simulink model "serialtest"  (Simulink 7.1)
settings: Solver=FixedStepDiscrete  StartTime=0.0  StopTime=10.0  RelTol=1e-3
values from neighbouring files (symbols this model uses):
  count = count+1    (= 2)    [findVI.m]
libraries: xpclib x4, simulink x1
settings Model: Creator=Administrator  LastModifiedBy=jporter  BufferReuse=off
settings DataIOCC: LimitDataPoints=off  SaveTime=off
settings OptimizationCC: BlockReduction=off  OptimizeBlockIOStorage=off  BufferReuse=off  ExpressionFolding=off  LocalBlockOutputs=off
settings HardwareCC: ProdIntDivRoundTo=Zero  ProdEndianess=LittleEndian  ProdHWDeviceType=Generic->32-bit x86 compatible
settings RTWCC: SystemTargetFile=xpctarget.tlc  TemplateMakefile=xpc_default_tmf  Description=xPC Target  ProcessScript=xpctarget_make_rtw_hook
settings xpcTargetCC: TargetFcnLib=ansi_tfl_table_tmw.mat  TargetFunctionLibrary=ANSI_C  CompOptLevelCompliant=off  PortableWordSizes=off  xPCisDownloadable=off

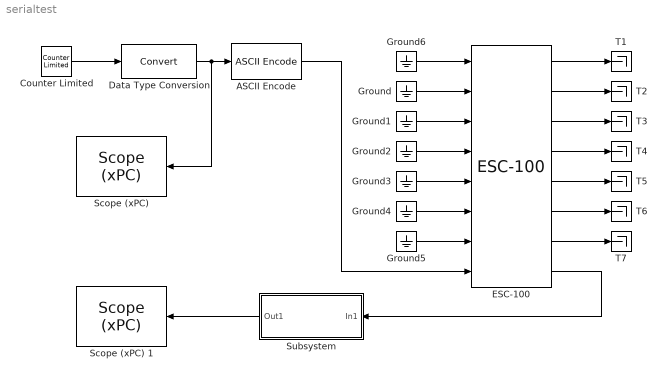
== system serialtest ==
  "ASCII Encode " : xpclib/RS232/ASCII Encode   format=%e\r  nvars=1  maxlength=128  vartypes={'double'}
  Counter Limited : simulink/Sources/Counter Limited  SystemSampleTime=-1  uplimit=99  tsamp=1
  Data Type Conversion : DataTypeConversion  OutDataType=sfix(16)  OutScaling=2^0
  ESC-100 : xpclib/RS232/Quatech/ESC-100/ESC-100  SystemSampleTime=-1  group=Basic Setup  port=8  irqnum=10  slot=[3,6]  baud1=9600  parity1=None  ndata1=8  nstop1=1  fifomode1=64 deep  rlevel1=1  automode1=on  xmtfifosize1=1024  xmtdatatype1=8 bit uint null terminated  rcvfifosize1=1024  rcvmaxread1=1024  rcvminread1=1  rcvusedelim1=on  rcvdelim1=13  rcvdatatype1=count+16 bit uint  rcvsampletime1=-1  baud2=115200  parity2=None  ndata2=8  nstop2=1  fifomode2=64 deep  rlevel2=half full  automode2=on  xmtfifosize2=1024  xmtdatatype2=8 bit uint null terminated  rcvfifosize2=1024  rcvmaxread2=1024  rcvminread2=1  rcvusedelim2=on  rcvdelim2=13  rcvdatatype2=count+16 bit uint  rcvsampletime2=-1  baud3=115200  parity3=None  ndata3=8  nstop3=1  fifomode3=64 deep  rlevel3=half full  automode3=on  xmtfifosize3=1024  xmtdatatype3=8 bit uint null terminated  rcvfifosize3=1024  rcvmaxread3=1024  rcvminread3=1  rcvusedelim3=on  rcvdelim3=13  rcvdatatype3=count+16 bit uint  rcvsampletime3=-1  buad4=115200  parity4=None  ndata4=8  nstop4=1  fifomode4=64 deep  rlevel4=half full  automode4=on  xmtfifosize4=1024  xmtdatatype4=8 bit uint null terminated  rcvfifosize4=1024  rcvmaxread4=1024  rcvminread4=1  rcvusedelim4=on  rcvdelim4=13  rcvdatatype4=count+16 bit uint  rcvsampletime4=-1  baud5=115200  parity5=None  ndata5=8  nstop5=1  fifomode5=64 deep  rlevel5=half full  automode5=on  xmtfifosize5=1024  xmtdatatype5=8 bit uint null terminated  rcvfifosize5=1024  rcvmaxread5=1024  rcvminread5=1  rcvusedelim5=on  rcvdelim5=13  rcvdatatype5=count+16 bit uint  rcvsampletime5=-1  baud6=115200  parity6=None  ndata6=8  nstop6=1  fifomode6=64 deep  rlevel6=half full  automode6=on  xmtfifosize6=1024  xmtdatatype6=8 bit uint null terminated  rcvfifosize6=1024  rcvmaxread6=1024  rcvminread6=1  rcvusedelim6=on  rcvdelim6=13  rcvdatatype6=count+16 bit uint  rcvsampletime6=-1  baud7=115200  parity7=None  ndata7=8  nstop7=1  fifomode7=64 deep  rlevel7=half full  automode7=on  xmtfifosize7=1024  xmtdatatype7=8 bit uint null terminated  rcvfifosize7=1024  rcvmaxread7=1024  rcvminread7=1  rcvusedelim7=on  rcvdelim7=13  rcvdatatype7=count+16 bit uint  rcvsampletime7=-1  baud8=9600  parity8=None  ndata8=8  nstop8=1  fifomode8=64 deep  rlevel8=quarter full  automode8=off  xmtfifosize8=1024  xmtdatatype8=8 bit uint null terminated  rcvfifosize8=1024  rcvmaxread8=16  rcvminread8=1  rcvusedelim8=off  rcvdelim8=13  rcvdatatype8=8 bit uint null terminated  rcvsampletime8=-1
  Ground{,1..6} (7 alike) : Ground
  "Scope (xPC) " : xpclib/Misc./Scope (xPC)   Orientation=left  SystemSampleTime=-1  scopeno=1  scopetype=Target  autostart=on  viewmode=Graphical sliding  formatstr='%15.6f'  grid=on  ylimits=[0,100]  nosamples=250  noprepostsamples=0  interleave=1  triggermode=FreeRun  triggersignal=1  triggerlevel=0.0  triggerslope=Either  triggerscope=1  triggersample=0  filename=data.dat  mode=Lazy  writesize=512  autorestart=off
  Scope (xPC) 1 : xpclib/Misc./Scope (xPC)   Orientation=left  SystemSampleTime=-1  scopeno=2  scopetype=Target  autostart=on  viewmode=Graphical sliding  formatstr='%15.6f'  grid=on  ylimits=[0,100]  nosamples=250  noprepostsamples=0  interleave=1  triggermode=FreeRun  triggersignal=1  triggerlevel=0.0  triggerslope=Either  triggerscope=1  triggersample=0  filename=data.dat  mode=Lazy  writesize=512  autorestart=off
  Subsystem : Subsystem  Orientation=left
  T{1..7} (7 alike) : Terminator
  wires:
  Counter Limited/1 -> Data Type Conversion/1
  Data Type Conversion/1 -> "ASCII Encode "/1, "Scope (xPC) "/1
  "ASCII Encode "/1 -> ESC-100/8
  ESC-100/1 -> T1/1
  ESC-100/2 -> T2/1
  ESC-100/3 -> T3/1
  ESC-100/4 -> T4/1
  ESC-100/5 -> T5/1
  ESC-100/6 -> T6/1
  ESC-100/7 -> T7/1
  Ground/1 -> ESC-100/2
  Ground1/1 -> ESC-100/3
  Ground2/1 -> ESC-100/4
  Ground3/1 -> ESC-100/5
  Ground4/1 -> ESC-100/6
  Ground5/1 -> ESC-100/7
  Ground6/1 -> ESC-100/1
  Subsystem/1(Out1) -> Scope (xPC) 1/1
  ESC-100/8 -> Subsystem/1(In1)

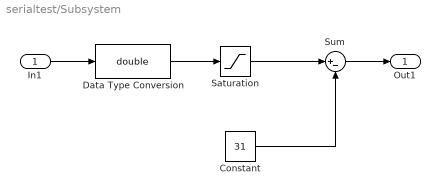
== system serialtest/Subsystem ==
  In1 : Inport  OutDataType=sfix(16)  OutScaling=2^0
  Constant : Constant  Value=31  OutDataType=sfix(16)  OutScaling=2^0
  Data Type Conversion : DataTypeConversion  OutDataTypeMode=double  OutDataType=sfix(16)  OutScaling=2^0  OutDataTypeStr=double  RndMeth=Nearest
  Saturation : Saturate  UpperLimit=127  LowerLimit=32  OutDataType=sfix(16)  OutScaling=2^0
  Sum : Sum  Inputs=|+-  OutDataType=sfix(16)  OutScaling=2^0
  Out1 : Outport  OutDataType=sfix(16)  OutScaling=2^0
  wires:
  In1/1 -> Data Type Conversion/1
  Data Type Conversion/1 -> Saturation/1
  Saturation/1 -> Sum/1
  Constant/1 -> Sum/2
  Sum/1 -> Out1/1
